simulink model "tracking_N_2015b"  (R2020a)
settings: Solver=VariableStepAuto  StartTime=0.0  StopTime=1000  RelTol=1e-3
InitFcn:
  | initdata
values from neighbouring files (symbols this model uses):
  A_siso = [-0.027023859725  0  0.0259844805048; 0  -0.0571658571106  0.0259844805048; 0.0259844805048  0.0259844805048  -0.0519689610096]    [control_1.mat]    (also in control_1_pertub.mat; control_1_perturb.mat; control_2.mat = [-0.0342183127648  0  0.0318309886184; 0  -0.0716197243914  ; control_2_perturb.mat = [-0.0342183127648  0  0.0318309886184; 0  -0.0716197243914  )
  B_siso = [0.00779534415144 0 0]    [control_1.mat]    (also in control_1_pertub.mat; control_1_perturb.mat; control_2.mat = [0.0159154943092 0 0]; control_2_perturb.mat = [0.0159154943092 0 0])
  K = [9.54000702209 -3.43386959649 -3.46052573093]    [control_1.mat]    (also in control_1_pertub.mat = [-3.54462170308 -6.57325869168 8.05083483607]; control_1_perturb.mat; control_2.mat = [13.3701574996 39.7393867777 42.5009231852]; control_2_perturb.mat = [13.3701574996 39.7393867777 42.5009231852])
  N = 25.8423310039    [control_1.mat]    (also in control_1_pertub.mat = 3.54019749053; control_1_perturb.mat; control_2.mat = -1.98186035374; control_2_perturb.mat = -1.98186035374)
settings Model: Creator=paulogil  LastModifiedBy=joaom
settings OptimizationCC: LifeSpan=inf
settings DebuggingCC: SFExecutionAtInitializationDiag=none  ArithmeticOperatorsInVariantConditions=warning
settings SFSimCC: CustomCodeUndefinedFunction=UseInterfaceOnly
settings CodeAppCC: StateflowObjectComments=on

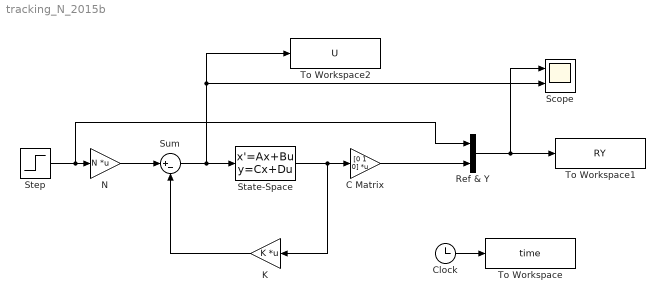
== system tracking_N_2015b ==
  C Matrix : Gain  Gain=[0 1 0]  Multiplication=Matrix(K*u)
  Clock : Clock
  K : Gain  Gain=K  Multiplication=Matrix(K*u)
  N : Gain  Gain=N  Multiplication=Matrix(K*u)
  Ref & Y : Mux  Inputs=2
  Scope : Scope  NumInputPorts=2
  State-Space : StateSpace  A=A_siso  B=B_siso*0.8  C=eye(3)  D=zeros(3,1)  InitialCondition=0
  Step : Step  Time=0  After=0.8  SampleTime=0
  Sum : Sum  Inputs=|+-
  To Workspace : ToWorkspace  VariableName=time  SaveFormat=Timeseries  SampleTime=-1
  To Workspace1 : ToWorkspace  VariableName=RY  SaveFormat=Timeseries  SampleTime=-1
  To Workspace2 : ToWorkspace  VariableName=U  SaveFormat=Timeseries  SampleTime=-1
  wires:
  State-Space/1 -> K/1, C Matrix/1
  Sum/1 -> To Workspace2/1, Scope/2, State-Space/1
  K/1 -> Sum/2
  N/1 -> Sum/1
  Step/1 -> Ref & Y/1, N/1
  C Matrix/1 -> Ref & Y/2
  Ref & Y/1 -> To Workspace1/1, Scope/1
  Clock/1 -> To Workspace/1
